simulink model "CircuitoProporcional"  (R2020a)
settings: Solver=VariableStepAuto  StartTime=0.0  StopTime=10.0  RelTol=1e-3
libraries: fl_lib x14
settings Model: Creator=matheusassis  LastModifiedBy=matheusassis
settings DebuggingCC: UnconnectedInputMsg=none  UnconnectedOutputMsg=none  UnconnectedLineMsg=none  SFMachineParentedDataDiag=error
settings ModelReferenceCC: EnableRefExpFcnMdlSchedulingChecks=off
settings RTWCC: Description=Generic Real-Time Target

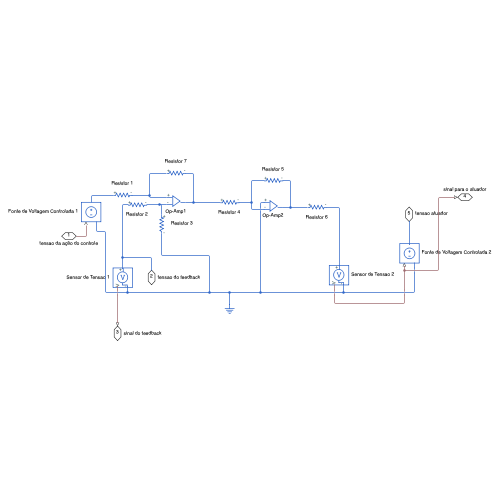
[thumbnail: Simulink's stored preview of the top-level diagram]
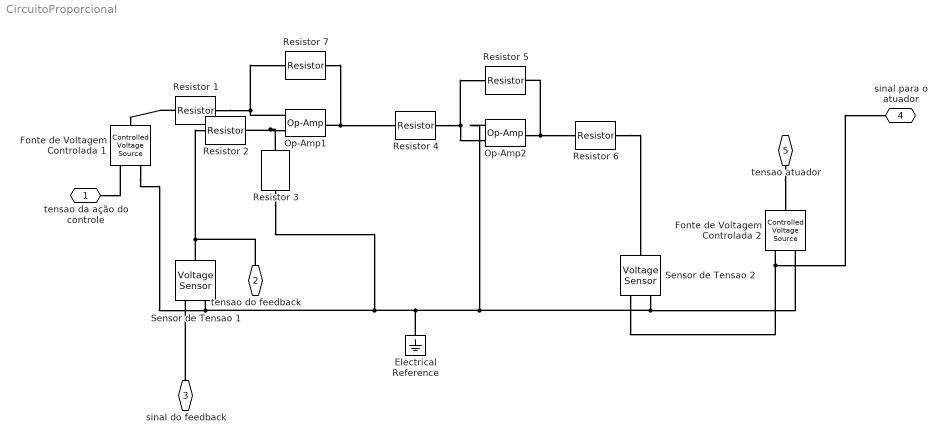
== system CircuitoProporcional ==
  Electrical Reference : fl_lib/Electrical/Electrical Elements/Electrical Reference
  Fonte de Voltagem Controlada 1 : fl_lib/Electrical/Electrical Sources/Controlled Voltage Source
  Fonte de Voltagem Controlada 2 : fl_lib/Electrical/Electrical Sources/Controlled Voltage Source
  Op-Amp1 : fl_lib/Electrical/Electrical Elements/Op-Amp  outI_specify=off  outI_priority=None  outI=0 A  outI_nominal_specify=off  outI_nominal_unit=A  outI_nominal_value=1
  Op-Amp2 : fl_lib/Electrical/Electrical Elements/Op-Amp  outI_specify=off  outI_priority=None  outI=0 A  outI_nominal_specify=off  outI_nominal_unit=A  outI_nominal_value=1
  Resistor {1..3,6..7} (5 alike) : fl_lib/Electrical/Electrical Elements/Resistor  R=1 Ohm  i_specify=off  i_priority=None  i=0 A  i_nominal_specify=off  i_nominal_unit=A  i_nominal_value=1  v_specify=off  v_priority=None  v=0 V  v_nominal_specify=off  v_nominal_unit=V  v_nominal_value=1
  Resistor 4 : fl_lib/Electrical/Electrical Elements/Resistor  R=10 Ohm  i_specify=off  i_priority=None  i=0 A  i_nominal_specify=off  i_nominal_unit=A  i_nominal_value=1  v_specify=off  v_priority=None  v=0 V  v_nominal_specify=off  v_nominal_unit=V  v_nominal_value=1
  Resistor 5 : fl_lib/Electrical/Electrical Elements/Resistor  R=3.4 Ohm  i_specify=off  i_priority=None  i=0 A  i_nominal_specify=off  i_nominal_unit=A  i_nominal_value=1  v_specify=off  v_priority=None  v=0 V  v_nominal_specify=off  v_nominal_unit=V  v_nominal_value=1
  Sensor de Tensao 1 : fl_lib/Electrical/Electrical Sensors/Voltage Sensor
  Sensor de Tensao 2 : fl_lib/Electrical/Electrical Sensors/Voltage Sensor
  tensao da ação do controle : PMIOPort  Side=Left
  tensao do feedback : PMIOPort  Port=2  Side=Left
  sinal do feedback : PMIOPort  Port=3  Side=Left
  sinal para o atuador : PMIOPort  Port=4  Side=Left
  tensao atuador : PMIOPort  Port=5  Side=Left
  connections:
  Resistor 1/LConn1 -- Fonte de Voltagem Controlada 1/LConn1
  Resistor 1/RConn1 -- Resistor 7/LConn1 -- Op-Amp1/LConn1
  Resistor 7/RConn1 -- Resistor 4/LConn1 -- Op-Amp1/RConn1
  Resistor 4/RConn1 -- Op-Amp2/LConn2 -- Resistor 5/LConn1
  Op-Amp2/RConn1 -- Resistor 6/LConn1 -- Resistor 5/RConn1
  Resistor 6/RConn1 -- Sensor de Tensao 2/LConn1
  Resistor 3/LConn1 -- Resistor 2/RConn1 -- Op-Amp1/LConn2
  Sensor de Tensao 1/LConn1 -- tensao do feedback/RConn1 -- Resistor 2/LConn1
  tensao da ação do controle/RConn1 -- Fonte de Voltagem Controlada 1/RConn1
  Sensor de Tensao 2/RConn2 -- Fonte de Voltagem Controlada 1/RConn2 -- Sensor de Tensao 1/RConn2 -- Resistor 3/RConn1 -- Electrical Reference/LConn1 -- Op-Amp2/LConn1 -- Fonte de Voltagem Controlada 2/RConn2
  sinal do feedback/RConn1 -- Sensor de Tensao 1/RConn1
  Sensor de Tensao 2/RConn1 -- sinal para o atuador/RConn1 -- Fonte de Voltagem Controlada 2/RConn1
  tensao atuador/RConn1 -- Fonte de Voltagem Controlada 2/LConn1
